simulink model "motorcontrol_codegen_19a"  (R2019a)
settings: Solver=FixedStepDiscrete  StartTime=0.0  StopTime=Inf  MaxStep=5e-5  RelTol=1e-3  EnableMultiTasking=on
values from neighbouring files (symbols this model uses):
  dataType = 'single'    [motorcontrol_codegen_params.m]
undefined symbols (not defined in the file or in its folder): ControlMode, ctrlParams, DiscIntNeverNeededParam, Down, GPTRIP1SEL, GPTRIP2SEL, inverter, mcb_isSimVar, NumBits1, NumBits2, PI_params, pmsm, Slope1, Slope2, Target, Ts, TZ1, TZ2, Up
libraries: simulink x14, c2802xlib x5, c2837xDlib x4, c280xlib x1, c2000lib x1
(part 2 of 3)

== system motorcontrol_codegen_19a/Motor_Control1/Input Scaling/ Calculate Position and Speed ==
  QEP_Position_Count : Inport
  QEP_Index_Latch : Inport  Port=2
  Offset : Inport  Port=3
  Data Store Write : DataStoreWrite  DataStoreName=EnClosedLoop
  Delay : Delay  DelayLength=1
  IndexFinder : Subsystem
  NOT : Logic  Operator=NOT  AllPortsSameDT=off  OutDataTypeStr=boolean
  Subsystem : Subsystem  mask{FilterConstant=0.01}
      mask prompts: FilterConstant "Filter coefficient"
      mask help:
      | Implement an IIR Filter on target hardware by implementing the formula:
      |
      |  y_k = a.x_k + (1-a).y_(k-1)
      |
      | Where, a is the filter coefficient.
      | Lower filter coefficient gives better filtering, but increases the delay in response time.
      mask TypeOptions FilterConstant: Filter_Constant/Value
      mask DialogControl DescGroupVar Prompt: IIR Filter
      mask DialogControl DescTextVar Prompt: Implement an IIR Filter on target hardware by implementing the formula:   y_k = a.x_k + (1-a).y_(k-1)  Where, a is the filter coefficient. Lower filter coefficient gives better filtering, but increases the delay in response time.
      mask Display: fprintf('IIR\n Filter')
  Subsystem1 : Subsystem  mask{DelayLength=16, SampleTimeAsync=Ts.pwm}
      mask prompts: DelayLength "Delays for speed calculation (number of samples):"; SampleTimeAsync "Block Sample Time (s):"
      mask DialogControl DescGroupVar Prompt: Speed Measurement
      mask DialogControl DescTextVar Prompt: Compute the speed from the rotor angular position. Output speed unit is RPM, input position unit is radians.
      mask Display:
      | color('black');
      | port_label('input' , 1 , '\theta' , 'texmode','on');
      | port_label('output',1,'\omega','texmode','on');
      | fprintf('Speed\n Measurement');
  Subsystem2 : Subsystem  mask(Quadrature Decoder){EncoderSlitsPerRevolution=pmsm.QEPSlits, EncoderCountsPerSlit=4, CounterSize=16 bits}
      mask prompts: EncoderSlitsPerRevolution "Encoder Slits:"; EncoderCountsPerSlit "Encoder counts per slit:"; CounterSize "Counter size:"
      mask help:
      | Compute the position of quadrature encoder.
      |
      | Cnt port accepts the quadrature encoder counter value. Idx port is enabled when the External index count is checked. Idx port accepts the counter value at last index pulse. The block only accepts scalar unsigned integer based on the Counter size parameter.
      mask TypeOptions CounterSize: 8 bits | 16 bits | 32 bits
      mask DialogControl DescTextVar Prompt: Compute the position of quadrature encoder.
      mask DialogControl Control2 Prompt: Cnt ports accepts the quadrature encoder counter value. Idx port is enabled when the external index count is checked. Idx port accepts the counter value at last index pulse. The block only accepts scalar unsigned integer based on the Counter size parameter.
      mask Display:
      | color('black');
      | port_label('input',1,'Cnt','interpreter','tex');
      | port_label('output',1,'\theta_m','interpreter','tex');
      | fprintf('Quadrature\nDecoder');
      | port_label('input',2,'Idx');
  Subsystem3 : Subsystem  mask{mechOffsetIn=0, maxAngleIn=2*pi, NrPP=pmsm.p}
      mask prompts: mechOffsetIn "Mechanical offset:"; maxAngleIn "Maximum input angle:"; NrPP "Number of pole pairs:"
      mask DialogControl DescGroupVar Prompt: Mechanical to Electrical Position
      mask DialogControl DescTextVar Prompt: Compute electrical position of the rotor based on mechanical position.
      mask Display:
      | port_label('input',1, '\theta_m','texmode','on');
      | port_label('input',2, 'Offset','texmode','on');
      | port_label('input',1, '\theta_e','texmode','on');
      | fprintf('Mech2Elec\n Position');
  Theta_e : Outport  VectorParamsAs1DForOutWhenUnconnected=off
  speed : Outport  Port=2  VectorParamsAs1DForOutWhenUnconnected=off
  IndexFound : Outport  Port=3  InitialOutput=0  VectorParamsAs1DForOutWhenUnconnected=off
  wires:
  QEP_Index_Latch/1 -> Subsystem2/2(IndexCount), IndexFinder/1(In1)
  IndexFinder/1(Out1) -> Delay/1, IndexFound/1, Data Store Write/1
  NOT/1 -> IndexFinder/Enable
  Delay/1 -> NOT/1
  Subsystem/1(y) -> speed/1
  Offset/1 -> Subsystem3/2(Offset)
  Subsystem2/1(Position) -> Subsystem1/1(Position), Subsystem3/1(ϴm)
  QEP_Position_Count/1 -> Subsystem2/1(Count)
  Subsystem3/1(ϴe) -> Theta_e/1
  Subsystem1/1(Speed) -> Subsystem/1(x)  "speed_meas"

== system motorcontrol_codegen_19a/Motor_Control1/Input Scaling/Calculate Phase Currents ==
  Ia_ADC : Inport
  Ib_ADC : Inport  Port=2
  Add : Sum  Inputs=-+
  Current Sense Gain : Gain  Gain=inverter.invertingAmp * inverter.I_max /(9.945)  RndMeth=Simplest  OutDataTypeStr=Inherit: Same as input
  Data Store Read1 : DataStoreRead  DataStoreName=IaOffset
  Data Store Read2 : DataStoreRead  DataStoreName=IbOffset
  Data Type Conversion : DataTypeConversion  OutDataTypeStr=int32  ConvertRealWorld=Stored Integer (SI)  RndMeth=Simplest
  Get_ADC_Volt : Gain  Gain=2048/12  OutDataTypeStr=dataType  RndMeth=Simplest
  Mux : Mux  Inputs=2
  Mux1 : Mux  Inputs=2
  Iab_meas : Outport  VectorParamsAs1DForOutWhenUnconnected=off
  wires:
  Current Sense Gain/1 -> Iab_meas/1
  Get_ADC_Volt/1 -> Current Sense Gain/1
  Mux1/1 -> Add/1
  Data Store Read2/1 -> Mux1/2
  Data Store Read1/1 -> Mux1/1
  Mux/1 -> Data Type Conversion/1
  Ib_ADC/1 -> Mux/2
  Ia_ADC/1 -> Mux/1
  Add/1 -> Get_ADC_Volt/1
  Data Type Conversion/1 -> Add/2

== system motorcontrol_codegen_19a/Motor_Control3/Control Modes/Position_Control ==
  note: The controller regulates motor position using rotor position feedback compared to a commanded position.
      | The output of the controller is the quadrature-winding current command which is directly proportional to the electromagnetic torque of the motor.
      | Since the motor being controlled is a Permanent Magnet Synchronous Machine, the rotor flux linkage is fixed (determined by the magnets),
      | hence the commanded direct-winding current is always zero.
  note: Position Controller
  position_command : Inport
  position_measured : Inport  Port=2
  Action Port : ActionPort  InitializeStates=reset
      settings: AttributesFormatString=----------------------------\nStates: %<InitializeStates>
  Isolate_For_Merge : SignalConversion  OverrideOpt=off
  Sum2 : Sum  Inputs=|+-
  q_current : Outport
  wires:
  position_measured/1 -> Sum2/2  "position_measured"
  position_command/1 -> Sum2/1  "position_command"
  Sum2/1 -> Isolate_For_Merge/1  "position_error"
  Isolate_For_Merge/1 -> q_current/1

== system motorcontrol_codegen_19a/Motor_Control3/Control Modes/Torque_Control ==
  note: The output of the controller is the quadrature-winding current command which is directly proportional to the electromagnetic torque of the motor.
      | In this configuration, the torque command is just the current command. An additional gain term could be added to translate current to torque
      | based on know motor parameters.
  note: Torque Controller
  torque_command : Inport
  Action Port : ActionPort
      settings: AttributesFormatString=----------------------------\nStates: %<InitializeStates>
  q_current : Outport
  wires:
  torque_command/1 -> q_current/1

== system motorcontrol_codegen_19a/Motor_Control3/Control Modes/Velocity_Control ==
  note: The controller regulates motor velocity using rotor velocity feedback compared to a commanded velocity.
      | The output of the controller is the quadrature-winding current command which is directly proportional to the electromagnetic torque of the motor.
      | Since the motor being controlled is a Permanent Magnet Synchronous Machine, the rotor flux linkage is fixed (determined by the magnets),
      | hence the commanded direct-winding current is always zero.
  note: Velocity Controller
  velocity_command : Inport
  velocity_measured : Inport  Port=2
  Action Port : ActionPort  InitializeStates=reset
      settings: AttributesFormatString=----------------------------\nStates: %<InitializeStates>
  Constant : Constant  Value=PI_params.Kp_speed  OutDataTypeStr=dataType  SampleTime=-1
  Constant1 : Constant  Value=PI_params.Ki_speed  OutDataTypeStr=dataType  SampleTime=-1
  Data Store Read1 : DataStoreRead  DataStoreName=Enable
  Isolate_For_Merge : SignalConversion  OverrideOpt=off
  Ki2 : Constant  Value=0  OutDataTypeStr=dataType  SampleTime=-1
  Logical Operator : Logic  Operator=NOT  IconShape=distinctive  AllPortsSameDT=off  OutDataTypeStr=boolean
  Rotor_Speed_Control : simulink/Continuous/PID Controller  Controller=PI  Form=Parallel  TimeDomain=Discrete-time  SampleTime=-1  IntegratorMethod=Forward Euler  FilterMethod=Forward Euler  ControllerParametersSource=external  P=ctrlParams.Velocity_P  I=ctrlParams.Velocity_I  D=0  UseFilter=on  N=100  TunerSelectOption=Transfer Function Based (PID Tuner App)  InitialConditionSource=external  InitialConditionForIntegrator=0  InitialConditionForFilter=0  DifferentiatorICPrevScaledInput=0  ExternalReset=level  TrackingMode=off  Kt=1  LimitOutput=on  UpperSaturationLimit=inverter.I_max  LowerSaturationLimit=-inverter.I_max  LinearizeAsGain=off  AntiWindupMode=clamping  Kb=0  POutMin=[]  POutMax=[]  IOutMin=[]  IOutMax=[]  DOutMin=[]  DOutMax=[]  NOutMin=[]  NOutMax=[]  SumOutMin=[]  SumOutMax=[]  SaturationOutMin=[]  SaturationOutMax=[]  PParamMin=[]  PParamMax=[]  IParamMin=[]  IParamMax=[]  DParamMin=[]  DParamMax=[]  NParamMin=[]  NParamMax=[]  KbParamMin=[]  KbParamMax=[]  KtParamMin=[]  KtParamMax=[]  KbOutMin=[]  KbOutMax=[]  KtOutMin=[]  KtOutMax=[]  IntegratorOutMin=[]  IntegratorOutMax=[]  FilterOutMin=[]  FilterOutMax=[]  SumI1OutMin=[]  SumI1OutMax=[]  SumI2OutMin=[]  SumI2OutMax=[]  SumI3OutMin=[]  SumI3OutMax=[]  SumI4OutMin=[]  SumI4OutMax=[]  SumDOutMin=[]  SumDOutMax=[]  DifferentiatorOutMin=[]  DifferentiatorOutMax=[]  FilterDiffOutCoefMin=[]  FilterDiffOutCoefMax=[]  ReciprocalOutMin=[]  ReciprocalOutMax=[]  SumDenOutMin=[]  SumDenOutMax=[]  SumNumOutMin=[]  SumNumOutMax=[]  DivideOutMin=[]  DivideOutMax=[]  IntegratorContinuousStateAttributes=''  IntegratorStateMustResolveToSignalObject=off  IntegratorRTWStateStorageClass=Auto  FilterContinuousStateAttributes=''  FilterStateMustResolveToSignalObject=off  FilterRTWStateStorageClass=Auto  ParallelPVariant=ExternalParameters  IdealPVariant=Disabled  IVariant=ExternalParameters  DVariant=Disabled  IntegratorVariant=Discrete  SatVariant=Enabled  AWVariant=DiscClampingParallel  PCopyVariant=Disabled  TRVariant=Disabled  FdbkBlocksVariant=Forward  IdealPFdbkVariant=Disabled  SatFdbkVariant=Disabled  DerivativeFilterVariant=Disabled  NVariant=Disabled  NCopyVariant=Disabled_SignalSpec  FilterICVariant=Disabled  IntegratorICVariant=ExternalICs  ExternalResetVariant=ExternalReset  TRSumVariant=Passthrough  SumFdbkVariant=Disabled  SumVariant=Sum_PI
  Sum2 : Sum  Inputs=|+-
  q_current : Outport
  wires:
  velocity_measured/1 -> Sum2/2  "velocity_measured"
  Sum2/1 -> Rotor_Speed_Control/1  "velocity_error"
  Rotor_Speed_Control/1 -> Isolate_For_Merge/1  "quadrature_current_command"
  velocity_command/1 -> Sum2/1  "velocity_command"
  Isolate_For_Merge/1 -> q_current/1
  Constant/1 -> Rotor_Speed_Control/2
  Constant1/1 -> Rotor_Speed_Control/3
  Data Store Read1/1 -> Logical Operator/1
  Logical Operator/1 -> Rotor_Speed_Control/4
  Ki2/1 -> Rotor_Speed_Control/5

== system motorcontrol_codegen_19a/Serial Receive/Simulation/Data_Type_Float ==
  In1 : Inport
  In2 : Inport  Port=2
  Data Type Conversion2 : DataTypeConversion  OutDataTypeStr=dataType  RndMeth=Simplest
  Mux : Mux  Inputs=2
  Data : Outport
  wires:
  Data Type Conversion2/1 -> Mux/2
  In2/1 -> Data Type Conversion2/1
  Mux/1 -> Data/1
  In1/1 -> Mux/1

== system motorcontrol_codegen_19a/Serial Receive/Simulation/Parse ==
  Enable_PWM : Inport
  Bitwise Operator : simulink/Logic and Bit Operations/Bitwise Operator  logicop=AND  UseBitMask=on  BitMask=hex2dec('0001')  BitMaskRealWorld=Stored Integer
  Data : Outport
  wires:
  Enable_PWM/1 -> Bitwise Operator/1
  Bitwise Operator/1 -> Data/1

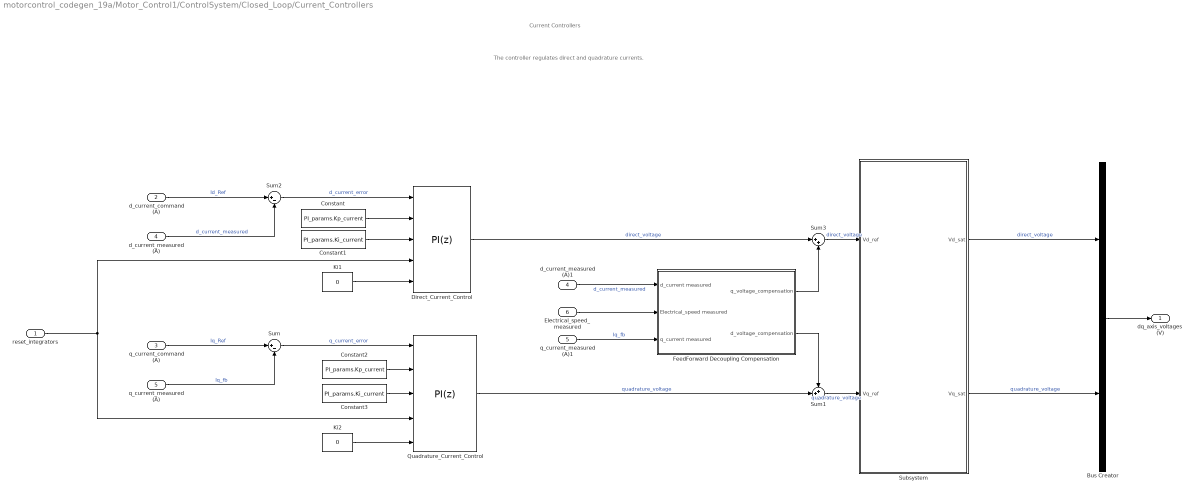
== system motorcontrol_codegen_19a/Motor_Control1/ControlSystem/Closed_Loop/Current_Controllers ==
  note: Current Controllers
  note: The controller regulates direct and quadrature currents.
  reset_integrators : Inport
  d_current_command (A) : Inport  Port=2
  q_current_command (A) : Inport  Port=3
  d_current_measured (A) : Inport  Port=4
  q_current_measured (A) : Inport  Port=5
  Electrical_speed_measured : Inport  Port=6
  Bus Creator : BusCreator  Inputs=2
  Constant : Constant  Value=PI_params.Kp_current  OutDataTypeStr=dataType  SampleTime=-1
  Constant1 : Constant  Value=PI_params.Ki_current  OutDataTypeStr=dataType  SampleTime=-1
  Constant2 : Constant  Value=PI_params.Kp_current  OutDataTypeStr=dataType  SampleTime=-1
  Constant3 : Constant  Value=PI_params.Ki_current  OutDataTypeStr=dataType  SampleTime=-1
  Direct_Current_Control : simulink/Continuous/PID Controller  Controller=PI  Form=Parallel  TimeDomain=Discrete-time  SampleTime=-1  IntegratorMethod=Forward Euler  FilterMethod=Forward Euler  ControllerParametersSource=external  P=ctrlParams.Current_P  I=ctrlParams.Current_I  D=0  UseFilter=on  N=100  TunerSelectOption=Transfer Function Based (PID Tuner App)  InitialConditionSource=external  InitialConditionForIntegrator=0  InitialConditionForFilter=0  DifferentiatorICPrevScaledInput=0  ExternalReset=level  TrackingMode=off  Kt=1  LimitOutput=on  UpperSaturationLimit=inverter.V_dc  LowerSaturationLimit=-inverter.V_dc  LinearizeAsGain=off  AntiWindupMode=clamping  Kb=0  POutMin=[]  POutMax=[]  IOutMin=[]  IOutMax=[]  DOutMin=[]  DOutMax=[]  NOutMin=[]  NOutMax=[]  SumOutMin=[]  SumOutMax=[]  SaturationOutMin=[]  SaturationOutMax=[]  PParamMin=[]  PParamMax=[]  IParamMin=[]  IParamMax=[]  DParamMin=[]  DParamMax=[]  NParamMin=[]  NParamMax=[]  KbParamMin=[]  KbParamMax=[]  KtParamMin=[]  KtParamMax=[]  KbOutMin=[]  KbOutMax=[]  KtOutMin=[]  KtOutMax=[]  IntegratorOutMin=[]  IntegratorOutMax=[]  FilterOutMin=[]  FilterOutMax=[]  SumI1OutMin=[]  SumI1OutMax=[]  SumI2OutMin=[]  SumI2OutMax=[]  SumI3OutMin=[]  SumI3OutMax=[]  SumI4OutMin=[]  SumI4OutMax=[]  SumDOutMin=[]  SumDOutMax=[]  DifferentiatorOutMin=[]  DifferentiatorOutMax=[]  FilterDiffOutCoefMin=[]  FilterDiffOutCoefMax=[]  ReciprocalOutMin=[]  ReciprocalOutMax=[]  SumDenOutMin=[]  SumDenOutMax=[]  SumNumOutMin=[]  SumNumOutMax=[]  DivideOutMin=[]  DivideOutMax=[]  IntegratorContinuousStateAttributes=''  IntegratorStateMustResolveToSignalObject=off  IntegratorRTWStateStorageClass=Auto  FilterContinuousStateAttributes=''  FilterStateMustResolveToSignalObject=off  FilterRTWStateStorageClass=Auto  ParallelPVariant=ExternalParameters  IdealPVariant=Disabled  IVariant=ExternalParameters  DVariant=Disabled  IntegratorVariant=Discrete  SatVariant=Enabled  AWVariant=DiscClampingParallel  PCopyVariant=Disabled  TRVariant=Disabled  FdbkBlocksVariant=Forward  IdealPFdbkVariant=Disabled  SatFdbkVariant=Disabled  DerivativeFilterVariant=Disabled  NVariant=Disabled  NCopyVariant=Disabled_SignalSpec  FilterICVariant=Disabled  IntegratorICVariant=ExternalICs  ExternalResetVariant=ExternalReset  TRSumVariant=Passthrough  SumFdbkVariant=Disabled  SumVariant=Sum_PI
      settings: AttributesFormatString=%<AntiWindupMode>
  FeedForward Decoupling Compensation : Subsystem
      mask Display: fprintf('Feed-forward \n Decoupling')
  Ki1 : Constant  Value=0  OutDataTypeStr=dataType  SampleTime=-1
  Ki2 : Constant  Value=0  OutDataTypeStr=dataType  SampleTime=-1
  Quadrature_Current_Control : simulink/Continuous/PID Controller  Controller=PI  Form=Parallel  TimeDomain=Discrete-time  SampleTime=-1  IntegratorMethod=Forward Euler  FilterMethod=Forward Euler  ControllerParametersSource=external  P=ctrlParams.Current_P  I=ctrlParams.Current_I  D=0  UseFilter=on  N=100  TunerSelectOption=Transfer Function Based (PID Tuner App)  InitialConditionSource=external  InitialConditionForIntegrator=0  InitialConditionForFilter=0  DifferentiatorICPrevScaledInput=0  ExternalReset=level  TrackingMode=off  Kt=1  LimitOutput=on  UpperSaturationLimit=inverter.V_dc  LowerSaturationLimit=-inverter.V_dc  LinearizeAsGain=off  AntiWindupMode=clamping  Kb=0  POutMin=[]  POutMax=[]  IOutMin=[]  IOutMax=[]  DOutMin=[]  DOutMax=[]  NOutMin=[]  NOutMax=[]  SumOutMin=[]  SumOutMax=[]  SaturationOutMin=[]  SaturationOutMax=[]  PParamMin=[]  PParamMax=[]  IParamMin=[]  IParamMax=[]  DParamMin=[]  DParamMax=[]  NParamMin=[]  NParamMax=[]  KbParamMin=[]  KbParamMax=[]  KtParamMin=[]  KtParamMax=[]  KbOutMin=[]  KbOutMax=[]  KtOutMin=[]  KtOutMax=[]  IntegratorOutMin=[]  IntegratorOutMax=[]  FilterOutMin=[]  FilterOutMax=[]  SumI1OutMin=[]  SumI1OutMax=[]  SumI2OutMin=[]  SumI2OutMax=[]  SumI3OutMin=[]  SumI3OutMax=[]  SumI4OutMin=[]  SumI4OutMax=[]  SumDOutMin=[]  SumDOutMax=[]  DifferentiatorOutMin=[]  DifferentiatorOutMax=[]  FilterDiffOutCoefMin=[]  FilterDiffOutCoefMax=[]  ReciprocalOutMin=[]  ReciprocalOutMax=[]  SumDenOutMin=[]  SumDenOutMax=[]  SumNumOutMin=[]  SumNumOutMax=[]  DivideOutMin=[]  DivideOutMax=[]  IntegratorContinuousStateAttributes=''  IntegratorStateMustResolveToSignalObject=off  IntegratorRTWStateStorageClass=Auto  FilterContinuousStateAttributes=''  FilterStateMustResolveToSignalObject=off  FilterRTWStateStorageClass=Auto  ParallelPVariant=ExternalParameters  IdealPVariant=Disabled  IVariant=ExternalParameters  DVariant=Disabled  IntegratorVariant=Discrete  SatVariant=Enabled  AWVariant=DiscClampingParallel  PCopyVariant=Disabled  TRVariant=Disabled  FdbkBlocksVariant=Forward  IdealPFdbkVariant=Disabled  SatFdbkVariant=Disabled  DerivativeFilterVariant=Disabled  NVariant=Disabled  NCopyVariant=Disabled_SignalSpec  FilterICVariant=Disabled  IntegratorICVariant=ExternalICs  ExternalResetVariant=ExternalReset  TRSumVariant=Passthrough  SumFdbkVariant=Disabled  SumVariant=Sum_PI
      settings: AttributesFormatString=%<AntiWindupMode>
  Subsystem : Subsystem  mask(DQ Limiter){Vmax=inverter.V_dc/sqrt(3)}
      mask prompts: Vmax "D-Q saturation limit:"
      mask help:
      | Implement saturation on reference dq voltages, with respect to phase voltage peak limit.
      |
      | The block accepts reference values of d and q axis voltages, and outputs corresponding saturated values along with unsaturated peak value to initiate field weakening control.
      |
      | Enter the phase voltage peak limit in the dialog box to initiate saturation.
      mask Display: fprintf('DQ Limiter');
  Sum : Sum  Inputs=|+-
  Sum1 : Sum  Inputs=++|
  Sum2 : Sum  Inputs=|+-
  Sum3 : Sum  Inputs=|++
  d_current_measured (A)1 : InportShadow  Port=4
  q_current_measured (A)1 : InportShadow  Port=5
  dq_axis_voltages (V) : Outport
  wires:
  Bus Creator/1 -> dq_axis_voltages (V)/1
  Sum2/1 -> Direct_Current_Control/1  "d_current_error"
  Sum/1 -> Quadrature_Current_Control/1  "q_current_error"
  reset_integrators/1 -> Quadrature_Current_Control/4, Direct_Current_Control/4
  d_current_measured (A)/1 -> Sum2/2  "d_current_measured"
  Quadrature_Current_Control/1 -> Sum1/2  "quadrature_voltage"
  FeedForward Decoupling Compensation/2(d_voltage_compensation) -> Sum1/1
  Direct_Current_Control/1 -> Sum3/1  "direct_voltage"
  FeedForward Decoupling Compensation/1(q_voltage_compensation) -> Sum3/2
  d_current_measured (A)1/1 -> FeedForward Decoupling Compensation/1(d_current measured)  "d_current_measured"
  q_current_measured (A)1/1 -> FeedForward Decoupling Compensation/3(q_current measured)  "Iq_fb"
  Electrical_speed_measured/1 -> FeedForward Decoupling Compensation/2(Electrical_speed measured)
  Subsystem/2(Vq_sat) -> Bus Creator/2  "quadrature_voltage"
  Subsystem/1(Vd_sat) -> Bus Creator/1  "direct_voltage"
  Sum3/1 -> Subsystem/1(Vd_ref)  "direct_voltage"
  Sum1/1 -> Subsystem/2(Vq_ref)  "quadrature_voltage"
  Constant/1 -> Direct_Current_Control/2
  Constant1/1 -> Direct_Current_Control/3
  Constant2/1 -> Quadrature_Current_Control/2
  Constant3/1 -> Quadrature_Current_Control/3
  Ki1/1 -> Direct_Current_Control/5
  Ki2/1 -> Quadrature_Current_Control/5
  d_current_command (A)/1 -> Sum2/1  "Id_Ref"
  q_current_command (A)/1 -> Sum/1  "Iq_Ref"
  q_current_measured (A)/1 -> Sum/2  "Iq_fb"

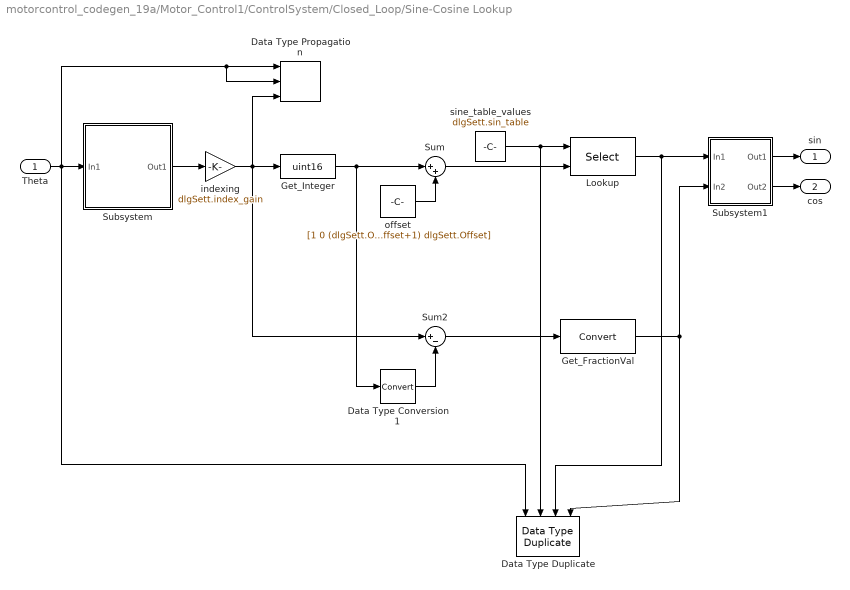
== system motorcontrol_codegen_19a/Motor_Control1/ControlSystem/Closed_Loop/Sine-Cosine Lookup ==
  Theta : Inport
  Data Type Duplicate : DataTypeDuplicate  NumInputPorts=4
  Data Type Propagation : simulink/Signal Attributes/Data Type Propagation  PropDataType=fixdt(1, 16)  IfRefDouble=double  IfRefSingle=single  IsSigned=IsSigned1 or IsSigned2  NumBitsBase=max([NumBits1 NumBits2])  NumBitsMult=1  NumBitsAdd=0  NumBitsAllowFinal=1:128  PropScalingMode=Obtain via best precision  PropScaling=2^-10  ValuesUsedBestPrec=[0 dlgSett.index_gain]  SlopeBase=min([Slope1 Slope2])  SlopeMult=1  SlopeAdd=0  BiasBase=Bias1  BiasMult=1  BiasAdd=0
      settings: SourceProductBaseCode=SL
  Data Type Conversion1 : DataTypeConversion  RndMeth=Simplest
  Get_FractionVal : DataTypeConversion  RndMeth=Simplest
  Get_Integer : DataTypeConversion  OutDataTypeStr=uint16  RndMeth=Simplest
  Lookup : Selector  IndexMode=Zero-based  InputPortWidth=dlgSett.size  IndexOptions=Index vector (port)  Indices=[1 3]  OutputSizes=1
  Subsystem : Subsystem
  Subsystem1 : Subsystem
  Sum : Sum  Inputs=|++  AccumDataTypeStr=uint32  OutDataTypeStr=uint32  RndMeth=Simplest
  Sum2 : Sum  Inputs=|+-  RndMeth=Simplest  OutDataTypeStr=Inherit: Same as first input
  indexing : Gain  Gain=dlgSett.index_gain  OutDataTypeStr=Inherit: Inherit via back propagation  RndMeth=Simplest
  offset : Constant  Value=[1 0 (dlgSett.Offset+1) dlgSett.Offset]  OutDataTypeStr=int16  SampleTime=-1
  sine_table_values : Constant  Value=dlgSett.sin_table  OutDataTypeStr=Inherit: Inherit via back propagation  SampleTime=-1
  sin : Outport  VectorParamsAs1DForOutWhenUnconnected=off
  cos : Outport  Port=2  VectorParamsAs1DForOutWhenUnconnected=off
  wires:
  Subsystem1/2(Out2) -> cos/1
  Data Type Conversion1/1 -> Sum2/2
  Subsystem1/1(Out1) -> sin/1
  offset/1 -> Sum/2
  Lookup/1 -> Subsystem1/1(In1), Data Type Duplicate/3
  Get_FractionVal/1 -> Subsystem1/2(In2), Data Type Duplicate/4
  Sum/1 -> Lookup/2
  Theta/1 -> Subsystem/1(In1), Data Type Propagation/1, Data Type Propagation/2, Data Type Duplicate/1
  indexing/1 -> Get_Integer/1, Data Type Propagation/3, Sum2/1
  sine_table_values/1 -> Data Type Duplicate/2, Lookup/1
  Get_Integer/1 -> Data Type Conversion1/1, Sum/1
  Sum2/1 -> Get_FractionVal/1
  Subsystem/1(Out1) -> indexing/1

== system motorcontrol_codegen_19a/Motor_Control1/ControlSystem/Closed_Loop/Subsystem ==
  note: D-Current Command
  note: The controller regulates motor velocity using rotor velocity feedback compared to a commanded velocity.
      | The output of the controller is the quadrature-winding current command which is directly proportional to the electromagnetic torque of the motor.
      | Since the motor being controlled is a Permanent Magnet Synchronous Machine, the rotor flux linkage is fixed (determined by the magnets),
      | hence the commanded direct-winding current is always zero.
  Zero : Constant  Value=0  OutDataTypeStr=dataType  SampleTime=-1
  d_current_command : Outport  OutDataTypeStr=dataType
  wires:
  Zero/1 -> d_current_command/1

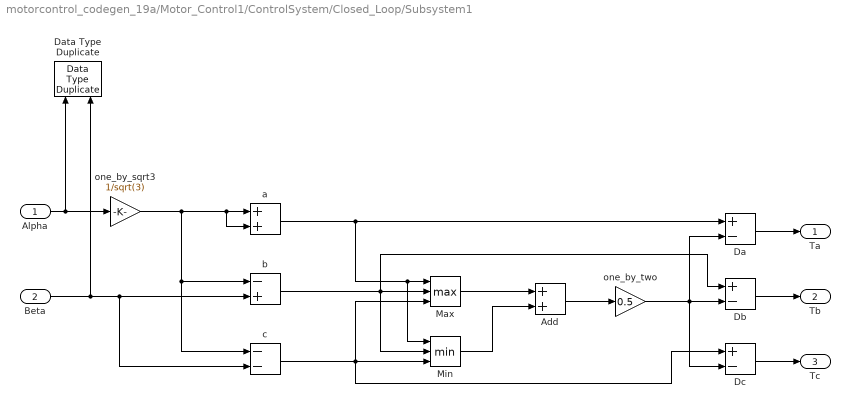
== system motorcontrol_codegen_19a/Motor_Control1/ControlSystem/Closed_Loop/Subsystem1 ==
  Alpha : Inport
  Beta : Inport  Port=2
  Add : Sum  RndMeth=Simplest  OutDataTypeStr=Inherit: Same as first input
  Da : Sum  Inputs=+-  RndMeth=Simplest  OutDataTypeStr=Inherit: Same as first input
  Data Type Duplicate : DataTypeDuplicate
  Db : Sum  Inputs=+-  RndMeth=Simplest  OutDataTypeStr=Inherit: Same as first input
  Dc : Sum  Inputs=+-  RndMeth=Simplest  OutDataTypeStr=Inherit: Same as first input
  Max : MinMax  Function=max  Inputs=3  RndMeth=Simplest
  Min : MinMax  Inputs=3  RndMeth=Simplest
  a : Sum  RndMeth=Simplest  OutDataTypeStr=Inherit: Same as first input
  b : Sum  Inputs=-+  RndMeth=Simplest  OutDataTypeStr=Inherit: Same as first input
  c : Sum  Inputs=--  RndMeth=Simplest  OutDataTypeStr=Inherit: Same as first input
  one_by_sqrt3 : Gain  Gain=1/sqrt(3)  RndMeth=Simplest  OutDataTypeStr=Inherit: Same as input  ParamDataTypeStr=Inherit: Same as input
  one_by_two : Gain  Gain=0.5  RndMeth=Simplest  OutDataTypeStr=Inherit: Same as input  ParamDataTypeStr=Inherit: Same as input
  Ta : Outport  VectorParamsAs1DForOutWhenUnconnected=off
  Tb : Outport  Port=2  VectorParamsAs1DForOutWhenUnconnected=off
  Tc : Outport  Port=3  VectorParamsAs1DForOutWhenUnconnected=off
  wires:
  Da/1 -> Ta/1
  a/1 -> Da/1, Min/1, Max/1
  Max/1 -> Add/1
  Dc/1 -> Tc/1
  Min/1 -> Add/2
  one_by_two/1 -> Dc/2, Db/2, Da/2
  Alpha/1 -> one_by_sqrt3/1, Data Type Duplicate/1
  one_by_sqrt3/1 -> c/1, b/1, a/2, a/1
  Db/1 -> Tb/1
  Beta/1 -> Data Type Duplicate/2, b/2, c/2
  Add/1 -> one_by_two/1
  c/1 -> Max/3, Dc/1, Min/3
  b/1 -> Db/1, Min/2, Max/2

== system motorcontrol_codegen_19a/Motor_Control1/ControlSystem/Closed_Loop/Subsystem2 ==
  a : Inport
  b : Inport  Port=2
  Data Type Duplicate : DataTypeDuplicate
  a_plus_2b : Sum  Inputs=+++  RndMeth=Simplest  OutDataTypeStr=Inherit: Same as first input
  one_by_sqrt3 : Gain  Gain=1/sqrt(3)  RndMeth=Simplest  OutDataTypeStr=Inherit: Same as input
  Alpha : Outport  VectorParamsAs1DForOutWhenUnconnected=off
  Beta : Outport  Port=2  VectorParamsAs1DForOutWhenUnconnected=off
  wires:
  a/1 -> a_plus_2b/1, Alpha/1, Data Type Duplicate/1
  a_plus_2b/1 -> one_by_sqrt3/1
  one_by_sqrt3/1 -> Beta/1
  b/1 -> a_plus_2b/2, a_plus_2b/3, Data Type Duplicate/2

== system motorcontrol_codegen_19a/Motor_Control1/ControlSystem/Closed_Loop/Subsystem3 ==
  Alpha : Inport
  Beta : Inport  Port=2
  sine : Inport  Port=3
  cos : Inport  Port=4
  Data Type Duplicate : DataTypeDuplicate  NumInputPorts=4
  Subsystem : Subsystem
  acos : Product  RndMeth=Simplest  OutDataTypeStr=Inherit: Same as first input
  asin : Product  RndMeth=Simplest  OutDataTypeStr=Inherit: Same as first input
  bcos : Product  OutDataTypeStr=Inherit: Inherit via back propagation  RndMeth=Simplest
  bsin : Product  OutDataTypeStr=Inherit: Inherit via back propagation  RndMeth=Simplest
  sum_Ds : Sum  Inputs=|++  RndMeth=Simplest  OutDataTypeStr=Inherit: Same as first input
  sum_Qs : Sum  Inputs=|+-  RndMeth=Simplest  OutDataTypeStr=Inherit: Same as first input
  Ds : Outport  VectorParamsAs1DForOutWhenUnconnected=off
  Qs : Outport  Port=2  VectorParamsAs1DForOutWhenUnconnected=off
  wires:
  Alpha/1 -> Data Type Duplicate/1, acos/1, asin/1
  acos/1 -> sum_Ds/1
  sine/1 -> bsin/2, asin/2, Data Type Duplicate/4
  asin/1 -> sum_Qs/2
  Subsystem/2(q_axis) -> Qs/1
  Beta/1 -> Data Type Duplicate/2, bcos/1, bsin/1
  sum_Qs/1 -> Subsystem/2(q)
  bsin/1 -> sum_Ds/2
  cos/1 -> Data Type Duplicate/3, bcos/2, acos/2
  bcos/1 -> sum_Qs/1
  Subsystem/1(d_axis) -> Ds/1
  sum_Ds/1 -> Subsystem/1(d)

== system motorcontrol_codegen_19a/Motor_Control1/ControlSystem/Closed_Loop/Subsystem4 ==
  Ds : Inport
  Qs : Inport  Port=2
  sin : Inport  Port=3
  cos : Inport  Port=4
  Data Type Duplicate : DataTypeDuplicate  NumInputPorts=4
  Subsystem : Subsystem
  dcos : Product  RndMeth=Simplest  OutDataTypeStr=Inherit: Same as first input
  dsin : Product  RndMeth=Simplest  OutDataTypeStr=Inherit: Same as first input
  qcos : Product  RndMeth=Simplest  OutDataTypeStr=Inherit: Same as first input
  qsin : Product  RndMeth=Simplest  OutDataTypeStr=Inherit: Same as first input
  sum_alpha : Sum  Inputs=|+-  RndMeth=Simplest  OutDataTypeStr=Inherit: Same as first input
  sum_beta : Sum  Inputs=|++  RndMeth=Simplest  OutDataTypeStr=Inherit: Same as first input
  Alpha : Outport  VectorParamsAs1DForOutWhenUnconnected=off
  Beta : Outport  Port=2  VectorParamsAs1DForOutWhenUnconnected=off
  wires:
  dsin/1 -> sum_beta/2
  sum_alpha/1 -> Subsystem/1(A)
  sin/1 -> Data Type Duplicate/4, qsin/2, dsin/2
  Subsystem/2(Beta) -> Beta/1
  Ds/1 -> Data Type Duplicate/1, dsin/1, dcos/1
  dcos/1 -> sum_alpha/1
  qcos/1 -> sum_beta/1
  sum_beta/1 -> Subsystem/2(B)
  Qs/1 -> Data Type Duplicate/2, qcos/1, qsin/1
  Subsystem/1(Alpha) -> Alpha/1
  qsin/1 -> sum_alpha/2
  cos/1 -> Data Type Duplicate/3, dcos/2, qcos/2

== system motorcontrol_codegen_19a/Motor_Control1/ControlSystem/Open Loop Start-Up/Ramp Generator ==
  Ramp_Time : Inport
  Enable : Inport  Port=2
  Divide : Product  Inputs=*/  RndMeth=Simplest  OutDataTypeStr=Inherit: Same as first input
  NOT : Logic  Operator=NOT  IconShape=distinctive  AllPortsSameDT=off  OutDataTypeStr=boolean
  One : Constant  OutDataTypeStr=dataType  SampleTime=-1
  Ramp Generator : DiscreteIntegrator  IntegratorMethod=Accumulation: Forward Euler  gainval=1  ExternalReset=sampled level  SampleTime=-1  OutDataTypeStr=dataType  RndMeth=Simplest  LimitOutput=on  UpperSaturationLimit=1  LowerSaturationLimit=0  ICPrevOutput=DiscIntNeverNeededParam  ICPrevScaledInput=DiscIntNeverNeededParam
  Sample_Time : Gain  Gain=Ts.pwm  RndMeth=Simplest  OutDataTypeStr=Inherit: Same as input
  Ramp : Outport
  wires:
  NOT/1 -> Ramp Generator/2
  Enable/1 -> NOT/1
  Ramp_Time/1 -> Divide/2
  One/1 -> Divide/1
  Sample_Time/1 -> Ramp Generator/1
  Ramp Generator/1 -> Ramp/1  "Eps"
  Divide/1 -> Sample_Time/1

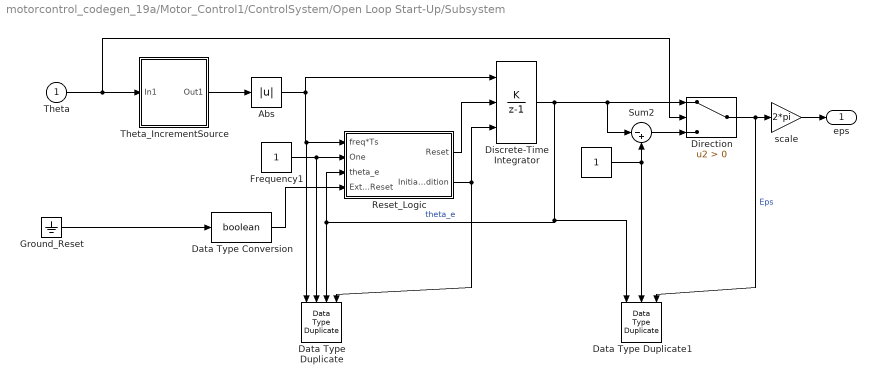
== system motorcontrol_codegen_19a/Motor_Control1/ControlSystem/Open Loop Start-Up/Subsystem ==
  Theta : Inport
  " " : Constant  OutDataTypeStr=Inherit: Inherit via back propagation  SampleTime=-1
  Abs : Abs
  Data Type Duplicate : DataTypeDuplicate  NumInputPorts=4
  Data Type Duplicate1 : DataTypeDuplicate  NumInputPorts=3
  Data Type Conversion : DataTypeConversion  OutDataTypeStr=boolean  RndMeth=Simplest
  Direction : Switch  Criteria=u2 > Threshold  OutDataTypeStr=Inherit: Inherit via back propagation  RndMeth=Simplest
  Discrete-Time Integrator : DiscreteIntegrator  IntegratorMethod=Accumulation: Forward Euler  ExternalReset=sampled level  InitialConditionSource=external  SampleTime=-1  OutDataTypeStr=Inherit: Inherit via back propagation  RndMeth=Simplest  LimitOutput=on  UpperSaturationLimit=1  LowerSaturationLimit=0  ICPrevOutput=DiscIntNeverNeededParam  ICPrevScaledInput=DiscIntNeverNeededParam
  Frequency1 : Constant  OutDataTypeStr=Inherit: Inherit via back propagation  SampleTime=-1
  Ground_Reset : Ground
  Reset_Logic : Subsystem
  Sum2 : Sum  Inputs=|-+  RndMeth=Simplest  OutDataTypeStr=Inherit: Same as first input
  Theta_IncrementSource : Subsystem
  scale : Gain  Gain=2*pi  RndMeth=Simplest  OutDataTypeStr=Inherit: Same as input
  eps : Outport  VectorParamsAs1DForOutWhenUnconnected=off
  wires:
  Reset_Logic/1(Reset) -> Discrete-Time Integrator/2
  Theta/1 -> Theta_IncrementSource/1(In1), Direction/2
  Frequency1/1 -> Reset_Logic/2(One), Data Type Duplicate/2
  Reset_Logic/2(Initial_Condition) -> Discrete-Time Integrator/3, Data Type Duplicate/4
  Theta_IncrementSource/1(Out1) -> Abs/1
  scale/1 -> eps/1
  Discrete-Time Integrator/1 -> Reset_Logic/3(theta_e), Data Type Duplicate/3, Data Type Duplicate1/1, Direction/1, Sum2/1  "theta_e"
  Sum2/1 -> Direction/3
  Abs/1 -> Reset_Logic/1(freq*Ts), Data Type Duplicate/1, Discrete-Time Integrator/1
  Ground_Reset/1 -> Data Type Conversion/1
  Direction/1 -> scale/1, Data Type Duplicate1/3  "Eps"
  " "/1 -> Data Type Duplicate1/2, Sum2/2
  Data Type Conversion/1 -> Reset_Logic/4(Extn_Reset)

== system motorcontrol_codegen_19a/Motor_Control1/ControlSystem/Open Loop Start-Up/Subsystem1 ==
  m : Inport
  Theta : Inport  Port=2
  Constant : Constant  Value=0  OutDataTypeStr=Inherit: Inherit via back propagation  SampleTime=-1
  Data Type Duplicate : DataTypeDuplicate  NumInputPorts=3
  Sine-Cosine Lookup : Subsystem  mask{N_points=1024}
      mask prompts: N_points "Number of data points for lookup table:"
      mask init: same as motorcontrol_codegen_19a/Motor_Control1/ControlSystem/Closed_Loop/Sine-Cosine Lookup
      mask DialogControl DescGroupVar Prompt: Sine-Cosine Lookup
      mask DialogControl DescTextVar Prompt: Implement sine and cosine functions using a lookup table approach for optimized performance on target hardware.
      mask Display: fprintf('Sin-Cos\n LUT');
  Subsystem1 : Subsystem  mask(Inverse Clarke Transform){}
      mask help:
      | <p>Compute Inverse Clarke transformation on balanced 2-phase orthogonal inputs into balanced 3-phase outputs.
      | <br><br>
      | The block accepts &alpha;-&beta; axis components and outputs corresponding 3-phase outputs, where phase-a axis is aligned with &alpha;-axis.</p>
      mask Display: fprintf('Inverse Clarke\n Transform');
  Subsystem2 : Subsystem  mask(Inverse Park Transform){AxisAlignment=D-axis}
      mask prompts: AxisAlignment "Alpha (phase-a ) axis alignment:"
      mask help:
      | <p>Compute Inverse Park transformation on rotating reference frame inputs into stationary reference frame outputs.
      | <br><br>
      | The block accepts the following:
      | <ul>
      | <li>d-q axis components in rotating reference frame</li>
      | <li>Sine and cosine values of corresponding angle of transformation</li>
      | </ul>
      | The block outputs &alpha;-&beta; axis components in stationary reference frame.
      | <br><br>
      | D-axis alignment with alpha (phase-a) is popular in motor control theory while Q-axis alignment with alpha (phase-a) is more suitable for power conversion applications.</p>
      mask init:
      | dlgSett.Offset = 0;
      | 
      | switch AxisAlignment
      |     case 'Q-axis'
      |         dlgSett.Offset = 90;
      |     case 'D-axis'
      |         dlgSett.Offset = 0;
      |     otherwise
      | end
      mask TypeOptions AxisAlignment: D-axis | Q-axis
      mask Display: fprintf('Inverse Park\n Transform');
  Unary Minus : UnaryMinus
  Va1 : Outport  VectorParamsAs1DForOutWhenUnconnected=off
  Vb1 : Outport  Port=2  VectorParamsAs1DForOutWhenUnconnected=off
  Vc1 : Outport  Port=3  VectorParamsAs1DForOutWhenUnconnected=off
  wires:
  Subsystem1/3(c) -> Vc1/1
  Subsystem2/1(Alpha) -> Subsystem1/1(In1)  "V_alpha"
  Theta/1 -> Sine-Cosine Lookup/1(Theta), Data Type Duplicate/2  "Eps"
  m/1 -> Unary Minus/1, Data Type Duplicate/1
  Unary Minus/1 -> Subsystem2/2(Qs)
  Subsystem2/2(Beta) -> Subsystem1/2(In2)  "V_beta"
  Subsystem1/1(a) -> Va1/1
  Subsystem1/2(b) -> Vb1/1
  Constant/1 -> Subsystem2/1(Ds), Data Type Duplicate/3
  Sine-Cosine Lookup/1(sin) -> Subsystem2/3(sin)
  Sine-Cosine Lookup/2(cos) -> Subsystem2/4(cos)

== system motorcontrol_codegen_19a/Motor_Control1/Input Scaling/ Calculate Position and Speed/IndexFinder ==
  In1 : Inport
  Enable : EnablePort
  AND : Logic  AllPortsSameDT=off  OutDataTypeStr=boolean
  Compare To Constant : simulink/Logic and Bit Operations/Compare To Constant  relop===  const=0  OutDataTypeStr=boolean
  Compare To Constant1 : simulink/Logic and Bit Operations/Compare To Constant  relop=>  const=0  OutDataTypeStr=boolean
  Delay3 : Delay  DelayLength=1
  Out1 : Outport
  wires:
  AND/1 -> Out1/1
  Delay3/1 -> Compare To Constant/1
  Compare To Constant/1 -> AND/1
  Compare To Constant1/1 -> AND/2
  In1/1 -> Compare To Constant1/1, Delay3/1

== system motorcontrol_codegen_19a/Motor_Control1/Input Scaling/ Calculate Position and Speed/Subsystem ==
  x : Inport
  Add : Sum
  Add1 : Sum  Inputs=-+
  Constant : Constant  OutDataTypeStr=single
  Data Type Duplicate : DataTypeDuplicate  NumInputPorts=3
  Filter_Constant : Constant  Value=FilterConstant  OutDataTypeStr=single
  Product : Product
  Product1 : Product
  Unit Delay : UnitDelay  SampleTime=-1  HasFrameUpgradeWarning=on
  y : Outport
  wires:
  x/1 -> Product/1, Data Type Duplicate/1
  Filter_Constant/1 -> Product/2, Add1/1, Data Type Duplicate/2
  Product/1 -> Add/1
  Add/1 -> y/1, Unit Delay/1
  Product1/1 -> Add/2
  Unit Delay/1 -> Product1/2
  Add1/1 -> Product1/1
  Constant/1 -> Data Type Duplicate/3, Add1/2

== system motorcontrol_codegen_19a/Motor_Control1/Input Scaling/ Calculate Position and Speed/Subsystem1 ==
  note: Speed measurement
  Position : Inport
  Delay : Delay  DelayLength=DelayLength  UseCircularBuffer=on
  SpeedCount : Sum  Inputs=+-|  OutDataTypeStr=int32  RndMeth=Simplest
  SpeedGain : Gain  Gain=single(2*pi)/(DelayLength*SampleTimeAsync(1)*4294967296)  ParamDataTypeStr=single  OutDataTypeStr=single  RndMeth=Simplest
  SpeedToCount : Gain  Gain=uint32(4294967296/6.2832)  ParamDataTypeStr=uint32  OutDataTypeStr=uint32  RndMeth=Simplest
  Speed : Outport  VectorParamsAs1DForOutWhenUnconnected=off
  wires:
  Position/1 -> SpeedToCount/1
  Delay/1 -> SpeedCount/2
  SpeedGain/1 -> Speed/1
  SpeedToCount/1 -> Delay/1, SpeedCount/1
  SpeedCount/1 -> SpeedGain/1

== system motorcontrol_codegen_19a/Motor_Control1/Input Scaling/ Calculate Position and Speed/Subsystem2 ==
  note: PositionComputation
  Count : Inport  OutDataTypeStr=uint16
  IndexCount : Inport  Port=2  OutDataTypeStr=uint16
  If1 : If
  Merge : Merge
  PositionGain : Gain  Gain=single(2*pi)/single(EncoderSlitsPerRevolution*4)  ParamDataTypeStr=single  OutDataTypeStr=single  RndMeth=Simplest
  PositionNoReset : Subsystem  TreatAsAtomicUnit=on
  PositionResetatIndex : Subsystem  TreatAsAtomicUnit=on
  ResetMode : Constant  OutDataTypeStr=int16
  Position : Outport  VectorParamsAs1DForOutWhenUnconnected=off
  wires:
  If1/2 -> PositionResetatIndex/Action
  If1/1 -> PositionNoReset/Action
  PositionGain/1 -> Position/1
  Merge/1 -> PositionGain/1
  ResetMode/1 -> If1/1
  PositionResetatIndex/1(Position) -> Merge/2
  Count/1 -> PositionNoReset/2(Count), PositionResetatIndex/1(Count)
  PositionNoReset/1(Position) -> Merge/1
  IndexCount/1 -> PositionNoReset/1(Index)

== system motorcontrol_codegen_19a/Motor_Control1/Input Scaling/ Calculate Position and Speed/Subsystem3 ==
  ϴm : Inport  OutMin=0  OutMax=maxAngleIn
  Offset : Inport  Port=2  OutMin=0  OutMax=1
  Data Type Duplicate : DataTypeDuplicate
  Subsystem : Subsystem
  Subsystem1 : Subsystem
  ϴe : Outport  VectorParamsAs1DForOutWhenUnconnected=off
  wires:
  Offset/1 -> Subsystem/2(In2)
  Subsystem1/2(ϴe) -> ϴe/1
  Subsystem1/1(Out1) -> Data Type Duplicate/2
  ϴm/1 -> Data Type Duplicate/1, Subsystem/1(ϴm)
  Subsystem/1(Out1) -> Subsystem1/1(In1)

== system motorcontrol_codegen_19a/Motor_Control1/ControlSystem/Closed_Loop/Current_Controllers/FeedForward Decoupling Compensation ==
  d_current measured : Inport
  Electrical_speed measured : Inport  Port=2
  q_current measured : Inport  Port=3
  Add : Sum
  Constant : Constant  Value=pmsm.Ld  OutDataTypeStr=Inherit: Inherit via back propagation  SampleTime=-1
  Constant1 : Constant  Value=pmsm.FluxPM  OutDataTypeStr=Inherit: Inherit via back propagation  SampleTime=-1
  Constant2 : Constant  Value=pmsm.Lq  OutDataTypeStr=Inherit: Inherit via back propagation  SampleTime=-1
  Data Type Duplicate : DataTypeDuplicate  NumInputPorts=6
  Product4 : Product  Inputs=3
  Product5 : Product
  Product6 : Product
  Unary Minus : UnaryMinus
  q_voltage_compensation : Outport
  d_voltage_compensation : Outport  Port=2
  wires:
  q_current measured/1 -> Product4/2, Data Type Duplicate/1
  Constant1/1 -> Data Type Duplicate/5, Add/2
  Product6/1 -> d_voltage_compensation/1
  Product4/1 -> Unary Minus/1
  Unary Minus/1 -> q_voltage_compensation/1
  Constant/1 -> Data Type Duplicate/4, Product5/2
  Product5/1 -> Add/1
  Electrical_speed measured/1 -> Product4/3, Product6/1, Data Type Duplicate/2
  Add/1 -> Product6/2
  d_current measured/1 -> Product5/1, Data Type Duplicate/3
  Constant2/1 -> Product4/1, Data Type Duplicate/6

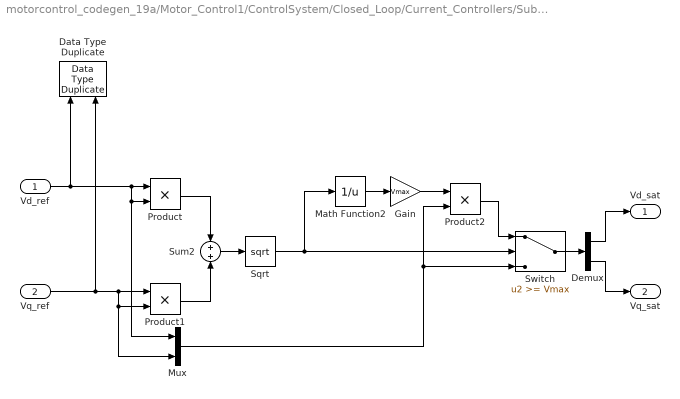
== system motorcontrol_codegen_19a/Motor_Control1/ControlSystem/Closed_Loop/Current_Controllers/Subsystem ==
  Vd_ref : Inport
  Vq_ref : Inport  Port=2
  Data Type Duplicate : DataTypeDuplicate
  Demux : Demux  Outputs=2
  Gain : Gain  Gain=Vmax  OutDataTypeStr=Inherit: Same as input
  Math Function2 : Math  Operator=reciprocal  RndMeth=Simplest
  Mux : Mux  Inputs=2
  Product : Product  RndMeth=Simplest  OutDataTypeStr=Inherit: Same as first input
  Product1 : Product  RndMeth=Simplest  OutDataTypeStr=Inherit: Same as first input
  Product2 : Product  OutDataTypeStr=Inherit: Same as first input
  Sqrt : Sqrt  IntermediateResultsDataTypeStr=Inherit: Inherit from input  SaturateOnIntegerOverflow=on
  Sum2 : Sum  OutDataTypeStr=Inherit: Same as first input
  Switch : Switch  Threshold=Vmax  ZeroCross=off
  Vd_sat : Outport  VectorParamsAs1DForOutWhenUnconnected=off
  Vq_sat : Outport  Port=2  VectorParamsAs1DForOutWhenUnconnected=off
  wires:
  Vd_ref/1 -> Mux/1, Product/2, Product/1, Data Type Duplicate/1
  Demux/1 -> Vd_sat/1
  Product1/1 -> Sum2/2
  Product/1 -> Sum2/1
  Sum2/1 -> Sqrt/1
  Gain/1 -> Product2/1
  Math Function2/1 -> Gain/1
  Vq_ref/1 -> Mux/2, Product1/2, Product1/1, Data Type Duplicate/2
  Mux/1 -> Switch/3, Product2/2
  Product2/1 -> Switch/1
  Demux/2 -> Vq_sat/1
  Sqrt/1 -> Switch/2, Math Function2/1
  Switch/1 -> Demux/1

== system motorcontrol_codegen_19a/Motor_Control1/ControlSystem/Closed_Loop/Sine-Cosine Lookup/Subsystem ==
  In1 : Inport
  Compare To Zero : simulink/Logic and Bit Operations/Compare To Zero  relop=<  OutDataTypeStr=boolean
  Data Type Conversion : DataTypeConversion  OutDataTypeStr=uint16  ConvertRealWorld=Stored Integer (SI)  RndMeth=Simplest
  If : If
  Merge : Merge
  Subsystem : Subsystem
  Subsystem1 : Subsystem
  convert_pu : Gain  Gain=1/(dlgSett.UpperSatLimit)  RndMeth=Simplest  OutDataTypeStr=Inherit: Same as input
  Out1 : Outport
  wires:
  If/2 -> Subsystem1/Action
  Subsystem/1(Out1) -> Merge/1
  convert_pu/1 -> Subsystem1/1(In1), Subsystem/1(In1), Compare To Zero/1
  In1/1 -> convert_pu/1
  If/1 -> Subsystem/Action
  Subsystem1/1(Out1) -> Merge/2
  Data Type Conversion/1 -> If/1
  Compare To Zero/1 -> Data Type Conversion/1
  Merge/1 -> Out1/1

== system motorcontrol_codegen_19a/Motor_Control1/ControlSystem/Closed_Loop/Sine-Cosine Lookup/Subsystem1 ==
  In1 : Inport
  In2 : Inport  Port=2
  Demux : Demux
  Product : Product  RndMeth=Simplest  OutDataTypeStr=Inherit: Same as first input
  Product1 : Product  RndMeth=Simplest  OutDataTypeStr=Inherit: Same as first input
  Sum3 : Sum  Inputs=|+-  RndMeth=Simplest  OutDataTypeStr=Inherit: Same as first input
  Sum4 : Sum  Inputs=|++  RndMeth=Simplest  OutDataTypeStr=Inherit: Same as first input
  Sum5 : Sum  Inputs=|+-  RndMeth=Simplest  OutDataTypeStr=Inherit: Same as first input
  Sum6 : Sum  Inputs=|++  RndMeth=Simplest  OutDataTypeStr=Inherit: Same as first input
  Out1 : Outport
  Out2 : Outport  Port=2
  wires:
  Sum4/1 -> Out1/1
  Sum5/1 -> Product1/1
  Sum6/1 -> Out2/1
  Demux/1 -> Sum3/1
  Demux/2 -> Sum4/2, Sum3/2
  Product/1 -> Sum4/1
  Sum3/1 -> Product/1
  Product1/1 -> Sum6/1
  Demux/4 -> Sum5/2, Sum6/2
  In1/1 -> Demux/1
  Demux/3 -> Sum5/1
  In2/1 -> Product1/2, Product/2

== system motorcontrol_codegen_19a/Motor_Control1/ControlSystem/Closed_Loop/Subsystem3/Subsystem ==
  d : Inport
  q : Inport  Port=2
  D_axis_aligned : Mux  Inputs=2
  Demux : Demux  Outputs=2
  Offset : Constant  Value=dlgSett.Offset  OutDataTypeStr=uint16  SampleTime=-1
  Q_axis_aligned : Mux  Inputs=2
  Switch : Switch  Criteria=u2 > Threshold  Threshold=1  RndMeth=Simplest  ZeroCross=off
  Unary_Minus : UnaryMinus
  d_axis : Outport  VectorParamsAs1DForOutWhenUnconnected=off
  q_axis : Outport  Port=2  VectorParamsAs1DForOutWhenUnconnected=off
  wires:
  d/1 -> D_axis_aligned/1, Q_axis_aligned/2
  Demux/1 -> d_axis/1
  Switch/1 -> Demux/1
  Offset/1 -> Switch/2
  D_axis_aligned/1 -> Switch/3
  q/1 -> D_axis_aligned/2, Unary_Minus/1
  Q_axis_aligned/1 -> Switch/1
  Demux/2 -> q_axis/1
  Unary_Minus/1 -> Q_axis_aligned/1

== system motorcontrol_codegen_19a/Motor_Control1/ControlSystem/Closed_Loop/Subsystem4/Subsystem ==
  A : Inport
  B : Inport  Port=2
  D_axis_aligned : Mux  Inputs=2
  Demux : Demux  Outputs=2
  Offset : Constant  Value=dlgSett.Offset  OutDataTypeStr=uint16  SampleTime=-1
  Q_axis_aligned : Mux  Inputs=2
  Switch : Switch  Criteria=u2 > Threshold  Threshold=1  RndMeth=Simplest  ZeroCross=off
  Unary_Minus : UnaryMinus
  Alpha : Outport  VectorParamsAs1DForOutWhenUnconnected=off
  Beta : Outport  Port=2  VectorParamsAs1DForOutWhenUnconnected=off
  wires:
  Q_axis_aligned/1 -> Switch/1
  Demux/1 -> Alpha/1
  D_axis_aligned/1 -> Switch/3
  Switch/1 -> Demux/1
  A/1 -> Unary_Minus/1, D_axis_aligned/1
  Demux/2 -> Beta/1
  B/1 -> Q_axis_aligned/1, D_axis_aligned/2
  Offset/1 -> Switch/2
  Unary_Minus/1 -> Q_axis_aligned/2

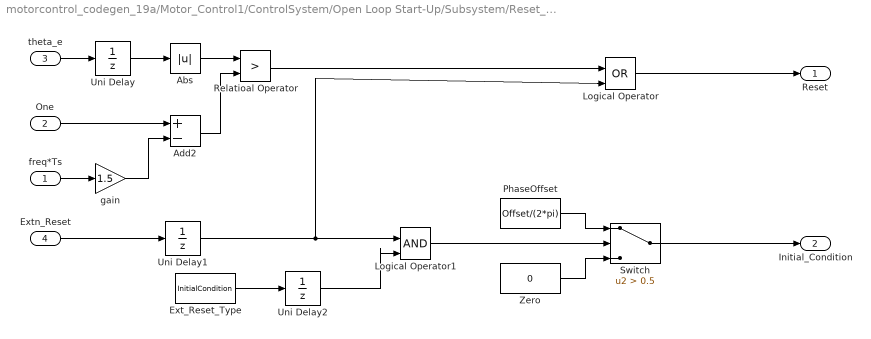
== system motorcontrol_codegen_19a/Motor_Control1/ControlSystem/Open Loop Start-Up/Subsystem/Reset_Logic ==
  freq*Ts : Inport
  One : Inport  Port=2
  theta_e : Inport  Port=3
  Extn_Reset : Inport  Port=4
  Abs : Abs  RndMeth=Simplest
  Add2 : Sum  Inputs=+-  RndMeth=Simplest  OutDataTypeStr=Inherit: Same as first input
  Ext_Reset_Type : Constant  Value=InitialCondition  OutDataTypeStr=boolean  SampleTime=-1
  Logical Operator : Logic  Operator=OR  IconShape=distinctive  AllPortsSameDT=off  OutDataTypeStr=boolean
  Logical Operator1 : Logic  IconShape=distinctive  AllPortsSameDT=off  OutDataTypeStr=boolean
  PhaseOffset : Constant  Value=Offset/(2*pi)  OutDataTypeStr=Inherit: Inherit via back propagation  SampleTime=-1
  Relatioal Operator : RelationalOperator  Operator=>  OutDataTypeStr=boolean  RndMeth=Simplest  InputSameDT=on
  Switch : Switch  Criteria=u2 > Threshold  Threshold=0.5  OutDataTypeStr=Inherit: Inherit via back propagation  RndMeth=Simplest
  Uni Delay : UnitDelay  SampleTime=-1  HasFrameUpgradeWarning=on
  Uni Delay1 : UnitDelay  InitialCondition=1  SampleTime=-1  HasFrameUpgradeWarning=on
  Uni Delay2 : UnitDelay  InitialCondition=1  SampleTime=-1  HasFrameUpgradeWarning=on
  Zero : Constant  Value=0  OutDataTypeStr=Inherit: Inherit via back propagation  SampleTime=-1
  gain : Gain  Gain=1.5  RndMeth=Simplest  OutDataTypeStr=Inherit: Same as input
  Reset : Outport  VectorParamsAs1DForOutWhenUnconnected=off
  Initial_Condition : Outport  Port=2  VectorParamsAs1DForOutWhenUnconnected=off
  wires:
  Uni Delay2/1 -> Logical Operator1/2
  theta_e/1 -> Uni Delay/1
  gain/1 -> Add2/2
  Logical Operator1/1 -> Switch/2
  Ext_Reset_Type/1 -> Uni Delay2/1
  freq*Ts/1 -> gain/1
  Logical Operator/1 -> Reset/1
  Uni Delay/1 -> Abs/1
  One/1 -> Add2/1
  Switch/1 -> Initial_Condition/1
  Relatioal Operator/1 -> Logical Operator/1
  Uni Delay1/1 -> Logical Operator/2, Logical Operator1/1
  Extn_Reset/1 -> Uni Delay1/1
  Add2/1 -> Relatioal Operator/2
  Zero/1 -> Switch/3
  PhaseOffset/1 -> Switch/1
  Abs/1 -> Relatioal Operator/1

== system motorcontrol_codegen_19a/Motor_Control1/ControlSystem/Open Loop Start-Up/Subsystem/Theta_IncrementSource ==
  In1 : Inport
  scale : Gain  Gain=1/(2*pi)  RndMeth=Simplest  OutDataTypeStr=Inherit: Same as input
  Out1 : Outport  VectorParamsAs1DForOutWhenUnconnected=off
  wires:
  In1/1 -> scale/1
  scale/1 -> Out1/1

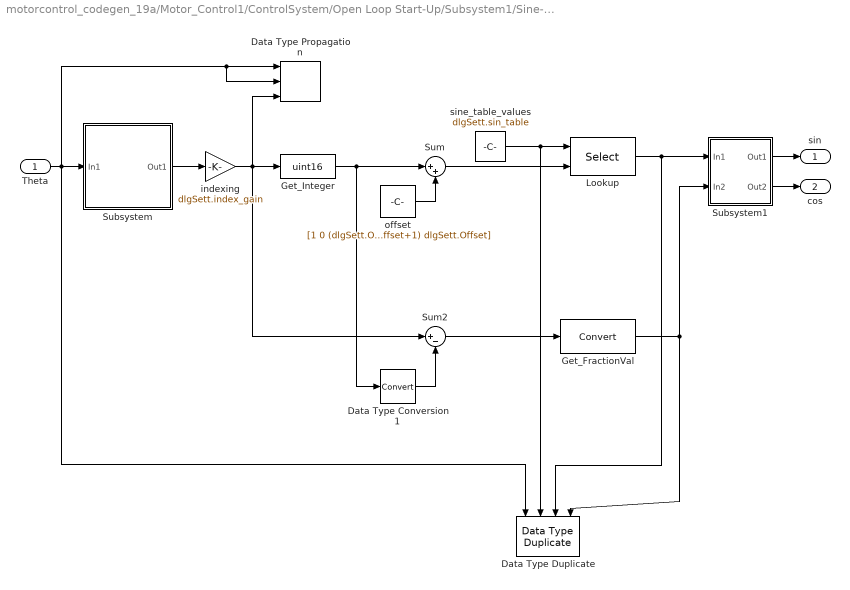
== system motorcontrol_codegen_19a/Motor_Control1/ControlSystem/Open Loop Start-Up/Subsystem1/Sine-Cosine Lookup ==
  Theta : Inport
  Data Type Duplicate : DataTypeDuplicate  NumInputPorts=4
  Data Type Propagation : simulink/Signal Attributes/Data Type Propagation  PropDataType=fixdt(1, 16)  IfRefDouble=double  IfRefSingle=single  IsSigned=IsSigned1 or IsSigned2  NumBitsBase=max([NumBits1 NumBits2])  NumBitsMult=1  NumBitsAdd=0  NumBitsAllowFinal=1:128  PropScalingMode=Obtain via best precision  PropScaling=2^-10  ValuesUsedBestPrec=[0 dlgSett.index_gain]  SlopeBase=min([Slope1 Slope2])  SlopeMult=1  SlopeAdd=0  BiasBase=Bias1  BiasMult=1  BiasAdd=0
      settings: SourceProductBaseCode=SL
  Data Type Conversion1 : DataTypeConversion  RndMeth=Simplest
  Get_FractionVal : DataTypeConversion  RndMeth=Simplest
  Get_Integer : DataTypeConversion  OutDataTypeStr=uint16  RndMeth=Simplest
  Lookup : Selector  IndexMode=Zero-based  InputPortWidth=dlgSett.size  IndexOptions=Index vector (port)  Indices=[1 3]  OutputSizes=1
  Subsystem : Subsystem
  Subsystem1 : Subsystem
  Sum : Sum  Inputs=|++  AccumDataTypeStr=uint32  OutDataTypeStr=uint32  RndMeth=Simplest
  Sum2 : Sum  Inputs=|+-  RndMeth=Simplest  OutDataTypeStr=Inherit: Same as first input
  indexing : Gain  Gain=dlgSett.index_gain  OutDataTypeStr=Inherit: Inherit via back propagation  RndMeth=Simplest
  offset : Constant  Value=[1 0 (dlgSett.Offset+1) dlgSett.Offset]  OutDataTypeStr=int16  SampleTime=-1
  sine_table_values : Constant  Value=dlgSett.sin_table  OutDataTypeStr=Inherit: Inherit via back propagation  SampleTime=-1
  sin : Outport  VectorParamsAs1DForOutWhenUnconnected=off
  cos : Outport  Port=2  VectorParamsAs1DForOutWhenUnconnected=off
  wires:
  Subsystem1/2(Out2) -> cos/1
  Data Type Conversion1/1 -> Sum2/2
  Subsystem1/1(Out1) -> sin/1
  offset/1 -> Sum/2
  Lookup/1 -> Subsystem1/1(In1), Data Type Duplicate/3
  Get_FractionVal/1 -> Subsystem1/2(In2), Data Type Duplicate/4
  Sum/1 -> Lookup/2
  Theta/1 -> Subsystem/1(In1), Data Type Propagation/1, Data Type Propagation/2, Data Type Duplicate/1
  indexing/1 -> Get_Integer/1, Data Type Propagation/3, Sum2/1
  sine_table_values/1 -> Data Type Duplicate/2, Lookup/1
  Get_Integer/1 -> Data Type Conversion1/1, Sum/1
  Sum2/1 -> Get_FractionVal/1
  Subsystem/1(Out1) -> indexing/1
